simulink model "Modelo_estrutura"  (R2015a)
settings: Solver=ode5  StartTime=0.0  StopTime=18  FixedStep=0.001  RelTol=1e-3
values from neighbouring files (symbols this model uses):
  A = [0,0,1,0;0,0,0,1;0,Ks/Ms,-Be*(Ms+Mc)/(Ms*Mc),0;0,-Ks/Ms,Be/Ms,0]    [Par_sistema_edif_amd.m]
  B = [0;0;K*(Ms+Mc)/(Mc*Ms);-K/Ms]    [Par_sistema_edif_amd.m]
  Be = (Kg^2*Kt^2)/(rmp^2*Rm)    (= 7.72356398165)    [Par_sistema_edif_amd.m]
  C = [1,0,0,0;0,-Ks/Ms,Be/Ms,0]    [Par_sistema_edif_amd.m]
  D = [0;-K/Ms]    [Par_sistema_edif_amd.m]
  K = Kg*Kt/(rmp*Rm)    (= 1.72354330709)    [Par_sistema_edif_amd.m]
  Ks = 500.8824    [Par_sistema_edif_amd.m]
  Mc = 0.65    [Par_sistema_edif_amd.m]
  Ms = 1.6    [Par_sistema_edif_amd.m]
settings Model: ExtModeTrigDuration=10000  Creator=Usuario  LastModifiedBy=Usuario
settings SolverCC: PositivePriorityOrder=on
settings RTWCC: SystemTargetFile=quarc_win64.tlc  TemplateMakefile=quarc_default_tmf  Description=QUARC Win64 Target
settings STFCustomTargetCC: TargetLibSuffix=.lib  TargetPreCompLibLocation=C:\PROGRA~3\QUARC\lib\2015a\win64\release  GenerateSampleERTMain=off  ConcurrentExecutionCompliant=on  GeneratePreprocessorConditionals=Disable all  ERTCustomFileBanners=off  SupportNonInlinedSFcns=on  SupportVariableSizeSignals=off  MATLABClassNameForMDSCustomization=Simulink.SoftwareTarget.GRTCustomization  GRTInterface=on  SystemTargetFile=quarc_win64.tlc
settings GRTTargetCC: TargetPreCompLibLocation=C:\PROGRA~3\QUARC\lib\2015a\win64\release  ParMdlRefBuildCompliant=off  CompOptLevelCompliant=off  CombineOutputUpdateFcns=off  MatFileLogging=off  CPPClassGenCompliant=off  GRTInterface=on  ExtMode=on  ExtModeMexFile=quarc_comm

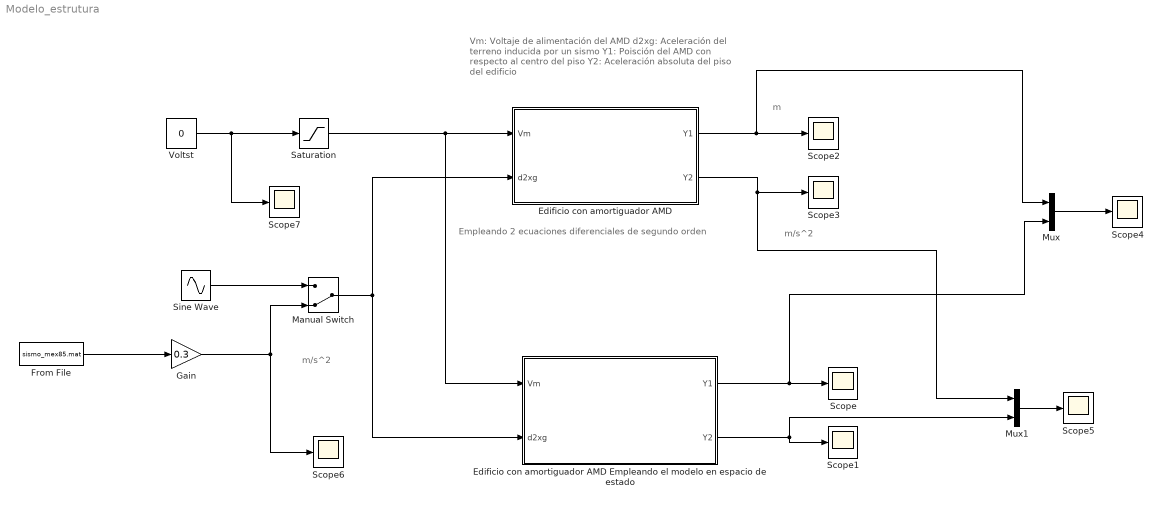
== system Modelo_estrutura ==
  note: m/s^2
  note: m
  note: m/s^2
  note: Empleando 2 ecuaciones diferenciales de segundo orden
  note: Vm: Voltaje de alimentación del AMD
      | d2xg: Aceleración del terreno inducida por un sismo
      | Y1: Poisción del AMD con respecto al centro del piso
      | Y2: Aceleración absoluta del piso del edificio
  Edificio con amortiguador AMD : Subsystem
  Edificio con amortiguador AMD Empleando el modelo en espacio de estado : Subsystem
  From File : FromFile  FileName=sismo_mex85.mat  SampleTime=0.001
  Gain : Gain  Gain=0.3
  Manual Switch : ManualSwitch  CurrentSetting=0
  Mux : Mux  Inputs=2
  Mux1 : Mux  Inputs=2
  Saturation : Saturate  UpperLimit=10  LowerLimit=-10
  Scope{,1..7} (8 alike) : Scope
      Scope2 settings: SaveName=ScopeData2
      Scope3 settings: SaveName=ScopeData3
      Scope4 settings: SaveName=ScopeData4
      Scope5 settings: SaveName=ScopeData5
      Scope6 settings: SaveName=ScopeData6
      Scope7 settings: SaveName=ScopeData7
  Sine Wave : Sin  SampleTime=0
  Voltst : Constant  Value=0
  wires:
  Sine Wave/1 -> Manual Switch/1
  Edificio con amortiguador AMD Empleando el modelo en espacio de estado/2(Y2) -> Mux1/2, Scope1/1
  Edificio con amortiguador AMD Empleando el modelo en espacio de estado/1(Y1) -> Mux/2, Scope/1
  Edificio con amortiguador AMD/1(Y1) -> Mux/1, Scope2/1
  Mux/1 -> Scope4/1
  Edificio con amortiguador AMD/2(Y2) -> Mux1/1, Scope3/1
  Mux1/1 -> Scope5/1
  Manual Switch/1 -> Edificio con amortiguador AMD/2(d2xg), Edificio con amortiguador AMD Empleando el modelo en espacio de estado/2(d2xg)
  From File/1 -> Gain/1
  Voltst/1 -> Scope7/1, Saturation/1
  Gain/1 -> Manual Switch/2, Scope6/1
  Saturation/1 -> Edificio con amortiguador AMD Empleando el modelo en espacio de estado/1(Vm), Edificio con amortiguador AMD/1(Vm)

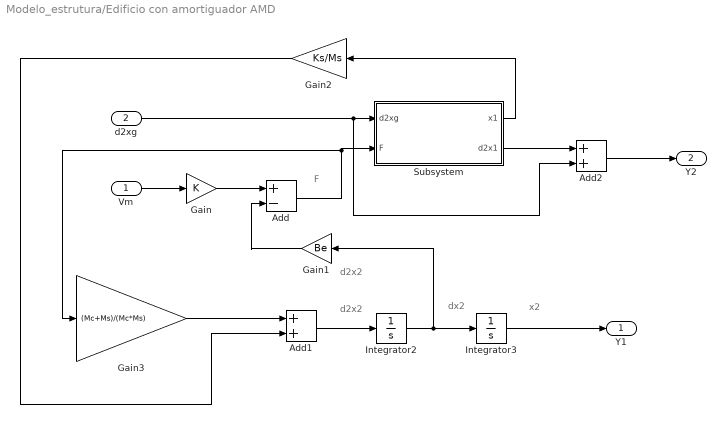
== system Modelo_estrutura/Edificio con amortiguador AMD ==
  note: d2x2
  note: F
  note: x2
  note: dx2
  note: d2x2
  Vm : Inport
  d2xg : Inport  Port=2
  Add : Sum  Inputs=+-
  Add1 : Sum
  Add2 : Sum
  Gain : Gain  Gain=K
  Gain1 : Gain  Gain=Be
  Gain2 : Gain  Gain=Ks/Ms
  Gain3 : Gain  Gain=(Mc+Ms)/(Mc*Ms)
  Integrator2 : Integrator
  Integrator3 : Integrator
  Subsystem : Subsystem
  Y1 : Outport
  Y2 : Outport  Port=2
  wires:
  Add2/1 -> Y2/1
  Subsystem/1(x1) -> Gain2/1
  Gain3/1 -> Add1/1
  Add1/1 -> Integrator2/1
  Integrator3/1 -> Y1/1
  Subsystem/2(d2x1) -> Add2/1
  Gain/1 -> Add/1
  Gain2/1 -> Add1/2
  d2xg/1 -> Subsystem/1(d2xg), Add2/2
  Add/1 -> Gain3/1, Subsystem/2(F)
  Vm/1 -> Gain/1
  Gain1/1 -> Add/2
  Integrator2/1 -> Gain1/1, Integrator3/1

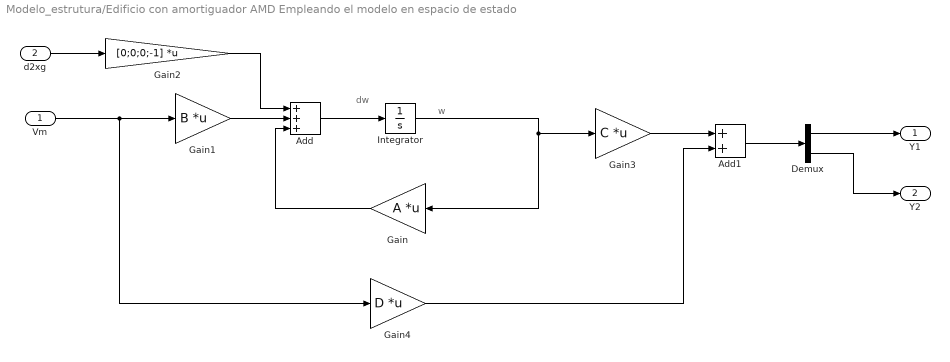
== system Modelo_estrutura/Edificio con amortiguador AMD Empleando el modelo en espacio de estado ==
  note: w
  note: dw
  Vm : Inport
  d2xg : Inport  Port=2
  Add : Sum  Inputs=+++
  Add1 : Sum
  Demux : Demux  Outputs=2
  Gain : Gain  Gain=A  Multiplication=Matrix(K*u)
  Gain1 : Gain  Gain=B  Multiplication=Matrix(K*u)
  Gain2 : Gain  Gain=[0;0;0;-1]  Multiplication=Matrix(K*u)
  Gain3 : Gain  Gain=C  Multiplication=Matrix(K*u)
  Gain4 : Gain  Gain=D  Multiplication=Matrix(K*u)
  Integrator : Integrator
  Y1 : Outport
  Y2 : Outport  Port=2
  wires:
  Integrator/1 -> Gain3/1, Gain/1
  Gain4/1 -> Add1/2
  Gain2/1 -> Add/1
  Add/1 -> Integrator/1
  Add1/1 -> Demux/1
  Gain3/1 -> Add1/1
  Demux/2 -> Y2/1
  Demux/1 -> Y1/1
  Gain1/1 -> Add/2
  Vm/1 -> Gain4/1, Gain1/1
  Gain/1 -> Add/3
  d2xg/1 -> Gain2/1

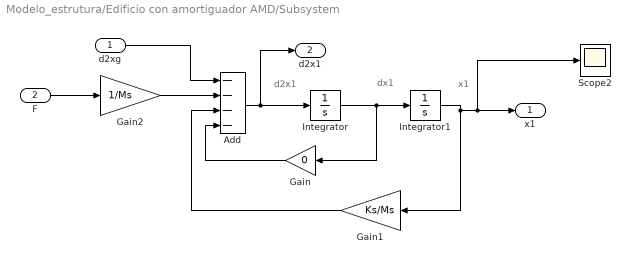
== system Modelo_estrutura/Edificio con amortiguador AMD/Subsystem ==
  note: x1
  note: dx1
  note: d2x1
  d2xg : Inport
  F : Inport  Port=2
  Add : Sum  Inputs=----
  Gain : Gain  Gain=0
  Gain1 : Gain  Gain=Ks/Ms
  Gain2 : Gain  Gain=1/Ms
  Integrator : Integrator
  Integrator1 : Integrator
  Scope2 : Scope
      settings: SaveName=ScopeData8
  x1 : Outport
  d2x1 : Outport  Port=2
  wires:
  Add/1 -> d2x1/1, Integrator/1
  Integrator/1 -> Gain/1, Integrator1/1
  Integrator1/1 -> Scope2/1, x1/1, Gain1/1
  Gain1/1 -> Add/3
  Gain2/1 -> Add/2
  F/1 -> Gain2/1
  Gain/1 -> Add/4
  d2xg/1 -> Add/1
